simulink model "usbSerialDataStream_Test"  (R2025b)
settings: Solver=FixedStepDiscrete  StartTime=0.0  StopTime=Inf  FixedStep=0.01  RelTol=1e-3
libraries: simulink x1, MagLevTbx_BaseLib x1
settings Model: ExtModeTrigDuration=2  Creator=riccardo  LastModifiedBy=riccardo
settings SolverCC: AutoInsertRateTranBlk=on
settings OptimizationCC: EnhancedBackFolding=on  PassReuseOutputArgsAs=Individual arguments  ZeroExternalMemoryAtStartup=off  ZeroInternalMemoryAtStartup=off  MaxStackSize=64  OptimizeBlockOrder=speed  DifferentSizesBufferReuse=on  OptimizationCustomize=off  EfficientTunableParamExpr=on
settings DebuggingCC: ParameterTunabilityLossMsg=error
settings HardwareCC: ProdBitPerPointer=32.0  ProdBitPerSizeT=32.0  ProdBitPerPtrDiffT=32.0  ProdLargestAtomicInteger=Long  ProdLargestAtomicFloat=Double  ProdWordSize=32.0  ProdHWDeviceType=ARM Compatible->ARM Cortex
settings SFSimCC: MATLABDynamicMemAlloc=off
settings RTWCC: SystemTargetFile=ert.tlc  HardwareBoard=Teensy 4.1 (Arduino Compatible)  TemplateMakefile=ert_default_tmf  Toolchain=Arduino ARM M7  BuildConfiguration=Faster Runs  Description=Embedded Coder
settings CodeAppCC: ForceParamTrailComments=on  IgnoreCustomStorageClasses=off  OperatorAnnotations=on  SimulinkDataObjDesc=on  SFDataObjDesc=on  InsertBlockDesc=on
settings ERTTargetCC: ExtModeTransport=3.0  ExtModeStaticAlloc=on  ExtModeAutomaticAllocSize=off  ExtModeStaticAllocSize=65536.0  ExtModeMexFile=ext_xcp  ExtModeIntrfLevel=Level2 - Open  InlinedParameterPlacement=Hierarchical  RootIOFormat=Structure reference  TargetLangStandard=C99 (ISO)  SupportContinuousTime=on  SupportVariableSizeSignals=on

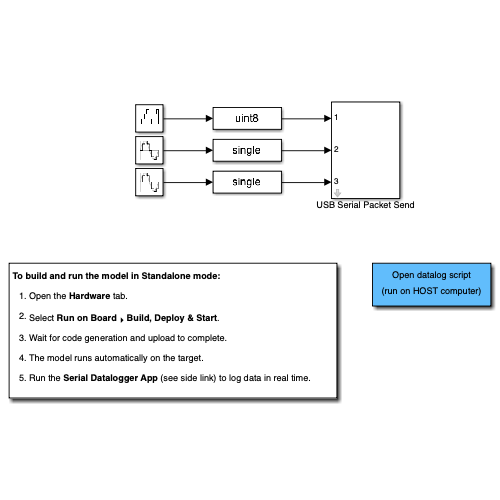
[thumbnail: Simulink's stored preview of the top-level diagram]
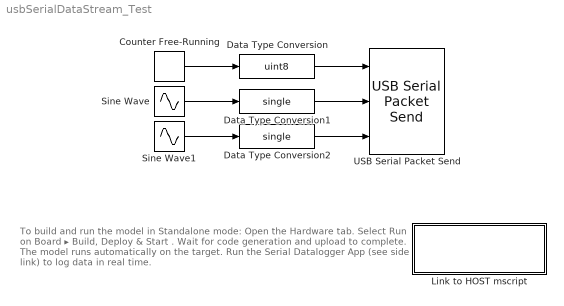
== system usbSerialDataStream_Test ==
  note: To build and run the model in Standalone mode:
      | Open the Hardware tab.
      | Select Run on Board ▸ Build, Deploy & Start .
      | Wait for code generation and upload to complete.
      | The model runs automatically on the target.
      | Run the Serial Datalogger App (see side link) to log data in real time.
  Counter Free-Running : simulink/Sources/Counter Free-Running  NumBits=8  tsamp=0.01
  Data Type Conversion : DataTypeConversion  OutDataTypeStr=uint8  SaturateOnIntegerOverflow=off  RndMeth=Floor
  Data Type Conversion1 : DataTypeConversion  OutDataTypeStr=single  SaturateOnIntegerOverflow=off  RndMeth=Floor
  Data Type Conversion2 : DataTypeConversion  OutDataTypeStr=single  SaturateOnIntegerOverflow=off  RndMeth=Floor
  Link to HOST mscript : Subsystem
      settings: OpenFcn=|
      | %  get toolbox base dir
      | info = MagLevTbx_Info();
      | 
      | %  path to HOST matlab script
      | mscriptpath = fullfile( ...
      | info.rootDir, ...
      | 'Examples', ...
      | 'UsbSerialDataStream_Test', ...
      | 'runSerialDataLoggerApp'  );
      | 
      | %  open script
      | edit( mscriptpath );
      | 
      | %  clear temp vars
      | clear info mscriptpath;
      mask Display:
      | disp(['Open datalog script\n\n' ...
      |     '(run on HOST computer)'])
  Sine Wave : Sin  Frequency=2*pi*1  SampleTime=0.01
  Sine Wave1 : Sin  Frequency=2*pi*1  Phase=pi/2  SampleTime=0.01
  USB Serial Packet Send : MagLevTbx_BaseLib/Communication/USB Serial Packet Send  waitDTR=on  packetSpec={'uint8', 'single', 'single'}  cobsEncoded=on  nullTerminated=on  sampleTime=-1  showEnablePort=off
      settings: SourceProductName=MagLev Toolbox
  wires:
  Counter Free-Running/1 -> Data Type Conversion/1
  Data Type Conversion/1 -> USB Serial Packet Send/1
  Data Type Conversion2/1 -> USB Serial Packet Send/3
  Data Type Conversion1/1 -> USB Serial Packet Send/2
  Sine Wave/1 -> Data Type Conversion1/1
  Sine Wave1/1 -> Data Type Conversion2/1

== system usbSerialDataStream_Test/Link to HOST mscript ==
